simulink model "diapo_blocks"  (R2014a)
settings: Solver=ode45  StartTime=0.0  StopTime=10.0  RelTol=1e-3
values from neighbouring files (symbols this model uses):
  L0 = 0.0015    [tipe_vars.m]
  Lbob = 0.06    [tipe_vars.m]
settings Model: Creator=jackhalford  LastModifiedBy=jackhalford
settings SolverCC: ShapePreserveControl=EnableAll  ZeroCrossControl=DisableAll

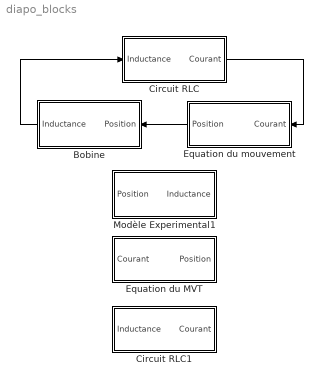
== system diapo_blocks ==
  Bobine : Subsystem
  Circuit RLC : Subsystem
  Circuit RLC1 : Subsystem
  Equation du MVT : Subsystem
  Equation du mouvement : Subsystem
  Modèle Experimental1 : Subsystem
  wires:
  Bobine/1(Inductance) -> Circuit RLC/1(Inductance)
  Equation du mouvement/1(Position) -> Bobine/1("Position ")
  Circuit RLC/1(Courant) -> Equation du mouvement/1(Courant)

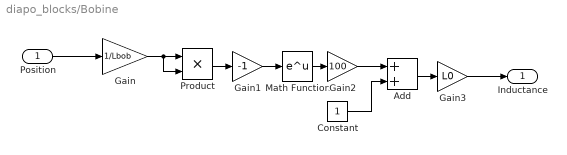
== system diapo_blocks/Bobine ==
  "Position " : Inport
  Add : Sum
  Constant : Constant
  Gain : Gain  Gain=1/Lbob
  Gain1 : Gain  Gain=-1
  Gain2 : Gain  Gain=100
  Gain3 : Gain  Gain=L0
  Math Function : Math  SaturateOnIntegerOverflow=on
  Product : Product
  Inductance : Outport
  wires:
  "Position "/1 -> Gain/1
  Gain/1 -> Product/2, Product/1
  Product/1 -> Gain1/1
  Gain1/1 -> Math Function/1
  Math Function/1 -> Gain2/1
  Gain2/1 -> Add/1
  Constant/1 -> Add/2
  Add/1 -> Gain3/1
  Gain3/1 -> Inductance/1

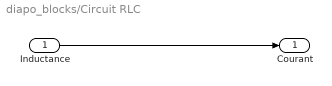
== system diapo_blocks/Circuit RLC ==
  Inductance : Inport
  Courant : Outport
  wires:
  Inductance/1 -> Courant/1

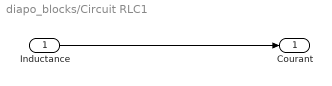
== system diapo_blocks/Circuit RLC1 ==
  Inductance : Inport
  Courant : Outport
  wires:
  Inductance/1 -> Courant/1

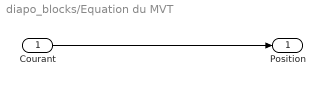
== system diapo_blocks/Equation du MVT ==
  Courant : Inport
  Position : Outport
  wires:
  Courant/1 -> Position/1

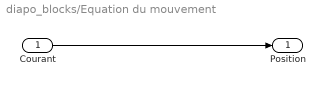
== system diapo_blocks/Equation du mouvement ==
  Courant : Inport
  Position : Outport
  wires:
  Courant/1 -> Position/1

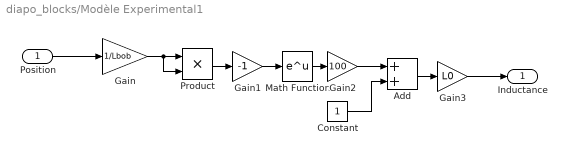
== system diapo_blocks/Modèle Experimental1 ==
  "Position " : Inport
  Add : Sum
  Constant : Constant
  Gain : Gain  Gain=1/Lbob
  Gain1 : Gain  Gain=-1
  Gain2 : Gain  Gain=100
  Gain3 : Gain  Gain=L0
  Math Function : Math  SaturateOnIntegerOverflow=on
  Product : Product
  Inductance : Outport
  wires:
  "Position "/1 -> Gain/1
  Gain/1 -> Product/2, Product/1
  Product/1 -> Gain1/1
  Gain1/1 -> Math Function/1
  Math Function/1 -> Gain2/1
  Gain2/1 -> Add/1
  Constant/1 -> Add/2
  Add/1 -> Gain3/1
  Gain3/1 -> Inductance/1
